simulink model "plt_aut"  (R2018b)
settings: Solver=ode45  StartTime=0.0  StopTime=5  MaxStep=0.01  RelTol=1e-3
values from neighbouring files (symbols this model uses):
  alpha = 1+1/(k*beta)    (= 1.025)    [tp1_syst_asservis.m]
  beta = 4    [tp1_syst_asservis.m]
  k = 10    [tp1_syst_asservis.m]
  to = 1.2    [tp1_syst_asservis.m]
settings Model: Creator=12210406  LastModifiedBy=12210406
settings DataIOCC: LimitDataPoints=on  SaveFormat=Array
settings OptimizationCC: BlockReduction=off  BooleanDataType=off  LifeSpan=inf
settings DebuggingCC: SaveWithParameterizedLinksMsg=none  UnderspecifiedInitializationDetection=Classic  MergeDetectMultiDrivingBlocksExec=none  SignalResolutionControl=TryResolveAllWithWarning  SFUnexpectedBacktrackingDiag=warning  SFNoUnconditionalDefaultTransitionDiag=warning  SFExecutionAtInitializationDiag=none
settings HardwareCC: ProdBitPerPointer=32  ProdBitPerSizeT=32  ProdBitPerPtrDiffT=32  ProdLargestAtomicFloat=None  ProdIntDivRoundTo=Undefined  ProdEndianess=Unspecified  ProdWordSize=32  ProdHWDeviceType=32-bit Generic  TargetUnknown=on
settings ModelReferenceCC: PropagateSignalLabelsOutOfModel=off
settings SFSimCC: SimUseLocalCustomCode=off
settings RTWCC: RTWUseLocalCustomCode=off
settings CodeAppCC: StateflowObjectComments=on
settings GRTTargetCC: TargetLangStandard=C89/C90 (ANSI)  GeneratePreprocessorConditionals=Disable all
settings ConfigComp: CovMetricSettings=dw  CovHtmlReporting=on  CovSaveCumulativeToWorkspaceVar=on  CovSaveSingleToWorkspaceVar=on  CovExternalEMLEnable=off  CovSFcnEnable=off

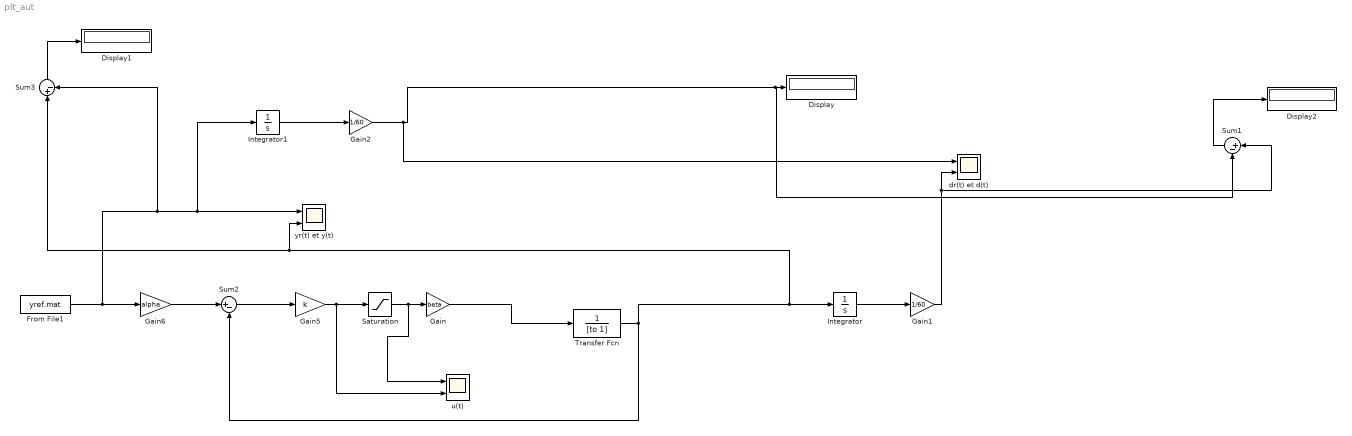
== system plt_aut ==
  Display : Display
  Display1 : Display
  Display2 : Display
  From File1 : FromFile  FileName=yref.mat  SampleTime=0
  Gain : Gain  Gain=beta
  Gain1 : Gain  Gain=1/60
  Gain2 : Gain  Gain=1/60
  Gain5 : Gain  Gain=k  ParamMax=[20]
  Gain6 : Gain  Gain=alpha
  Integrator : Integrator  UpperSaturationLimit=t  LowerSaturationLimit=0
  Integrator1 : Integrator  UpperSaturationLimit=t  LowerSaturationLimit=0
  Saturation : Saturate  UpperLimit=100  LowerLimit=-50
  Sum1 : Sum  Inputs=|+-
  Sum2 : Sum  Inputs=|+-
  Sum3 : Sum  Inputs=|+-
  Transfer Fcn : TransferFcn  Denominator=[to 1]
  dr(t) et d(t) : Scope  NumInputPorts=2
  u(t) : Scope  NumInputPorts=2
  yr(t) et y(t) : Scope  NumInputPorts=2
  wires:
  Transfer Fcn/1 -> Sum3/1, yr(t) et y(t)/2, Integrator/1, Sum2/2
  Integrator/1 -> Gain1/1
  Saturation/1 -> u(t)/1, Gain/1
  Gain6/1 -> Sum2/1
  Sum2/1 -> Gain5/1
  Gain5/1 -> u(t)/2, Saturation/1
  Integrator1/1 -> Gain2/1
  Gain2/1 -> dr(t) et d(t)/1, Sum1/2, Display/1
  From File1/1 -> Sum3/2, Integrator1/1, yr(t) et y(t)/1, Gain6/1
  Gain1/1 -> Sum1/1, dr(t) et d(t)/2
  Sum3/1 -> Display1/1
  Gain/1 -> Transfer Fcn/1
  Sum1/1 -> Display2/1
